simulink model "Vehicle_trailer_FreeModelControl_Modified"  (Simulink 7.7)
settings: Solver=ode3  StartTime=0.0  StopTime=50  FixedStep=Ts  RelTol=1e-3
undefined symbols (not defined in the file): alfa1, BWbaja, Df, jkk, kdf, kif, kpf, L1, L12, L2, manuever, tolerance, v
libraries: simulink x1
settings Model: Creator=Sara  LastModifiedBy=Raul
settings DataIOCC: SignalLoggingSaveFormat=Dataset
settings OptimizationCC: ExpressionDepthLimit=128
settings DebuggingCC: UnderspecifiedInitializationDetection=Simplified  MergeDetectMultiDrivingBlocksExec=error  SolverPrmCheckMsg=none  FcnCallInpInsideContextMsg=Enable All  StateNameClashWarn=none
settings CodeAppCC: CustomSymbolStrType=$N$R$M_T
settings GRTTargetCC: TargetFunctionLibrary=C89/C90 (ANSI)

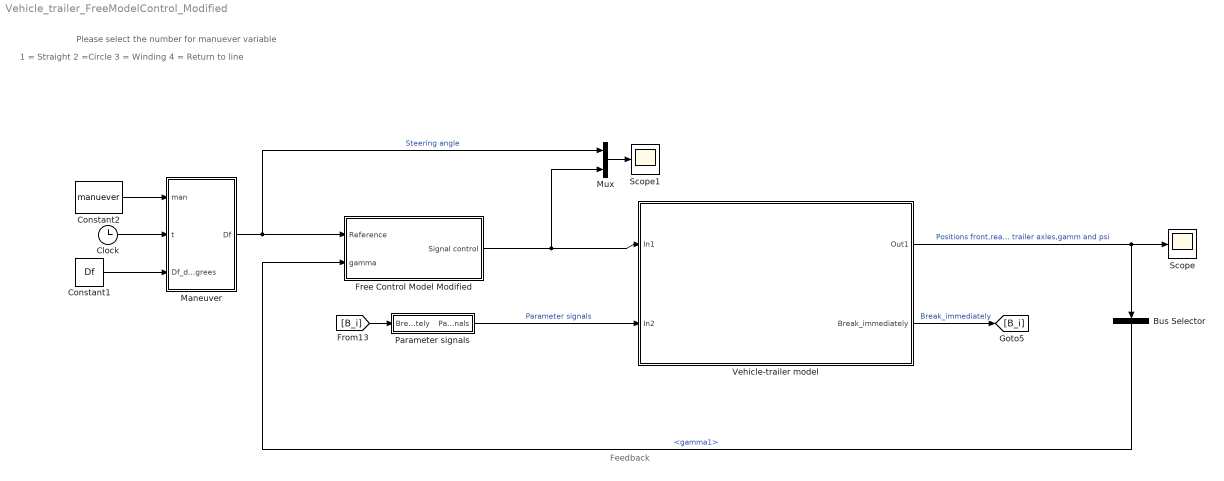
== system Vehicle_trailer_FreeModelControl_Modified ==
  note: 1 = Straight
      | 2 =Circle
      | 3 = Winding
      | 4 = Return to line
  note: Please select the number for manuever variable
  note: Feedback
  Bus Selector : BusSelector  OutputSignals=gamma1
  Clock : Clock
      settings: Decimation=10
  Constant1 : Constant  Value=Df
  Constant2 : Constant  Value=manuever
  Free Control Model Modified : Subsystem
  Maneuver : Stateflow chart  TreatAsAtomicUnit=on
  Mux : Mux  Inputs=2
  Parameter signals : Subsystem
  Scope : Scope
      settings: YMin=-15.4299  YMax=114.11
  Scope1 : Scope
      settings: YMin=-1  YMax=1  SaveName=ScopeData_SteeringAngle
  Vehicle-trailer model : Subsystem
      mask Display: image(imread('vt.png'))
  wires:
  Maneuver/1(Df) -> Mux/1, Free Control Model Modified/1(Reference)  "Steering angle"
  Constant2/1 -> Maneuver/1(man)
  Clock/1 -> Maneuver/2(t)
  Parameter signals/1(Parameter signals) -> Vehicle-trailer model/2(In2)  "Parameter signals"
  Vehicle-trailer model/2(Break_immediately) -> [B_i]  "Break_immediately"
  [B_i] -> Parameter signals/1(Break_immediately)
  Constant1/1 -> Maneuver/3(Df_degrees)
  Free Control Model Modified/1(Signal control) -> Vehicle-trailer model/1(In1), Mux/2
  Bus Selector/1 -> Free Control Model Modified/2(gamma)  "<gamma1>"
  Mux/1 -> Scope1/1
  Vehicle-trailer model/1(Out1) -> Scope/1, Bus Selector/1  "Positions front,rear and trailer axles,gamm and psi"

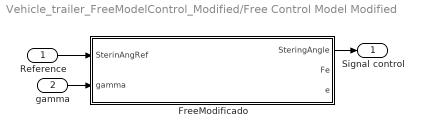
== system Vehicle_trailer_FreeModelControl_Modified/Free Control Model Modified ==
  Reference : Inport
  gamma : Inport  Port=2
  FreeModificado : Subsystem
  Signal control : Outport
  wires:
  Reference/1 -> FreeModificado/1(SterinAngRef)
  FreeModificado/1(SteringAngle) -> Signal control/1
  gamma/1 -> FreeModificado/2(gamma)

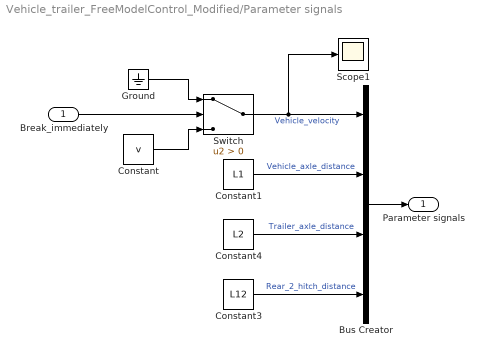
== system Vehicle_trailer_FreeModelControl_Modified/Parameter signals ==
  Break_immediately : Inport
  Bus Creator : BusCreator
  Constant : Constant  Value=v
  Constant1 : Constant  Value=L1
  Constant3 : Constant  Value=L12
  Constant4 : Constant  Value=L2
  Ground : Ground
  Scope1 : Scope
      settings: YMin=-1  YMax=1  SaveName=ScopeData4
  Switch : Switch  Criteria=u2 > Threshold
  Parameter signals : Outport
  wires:
  Constant1/1 -> Bus Creator/2  "Vehicle_axle_distance"
  Constant4/1 -> Bus Creator/3  "Trailer_axle_distance"
  Constant3/1 -> Bus Creator/4  "Rear_2_hitch_distance"
  Bus Creator/1 -> Parameter signals/1
  Switch/1 -> Bus Creator/1, Scope1/1  "Vehicle_velocity"
  Break_immediately/1 -> Switch/2
  Ground/1 -> Switch/1
  Constant/1 -> Switch/3

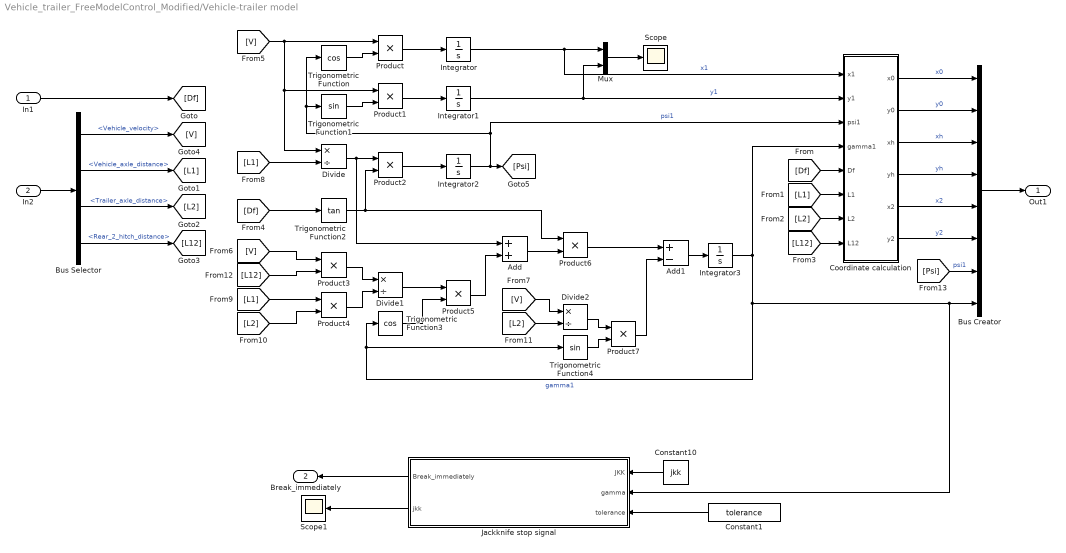
== system Vehicle_trailer_FreeModelControl_Modified/Vehicle-trailer model ==
  In1 : Inport
  In2 : Inport  Port=2
  Add : Sum
  Add1 : Sum  Inputs=+-
  Bus Creator : BusCreator  Inputs=8
  Bus Selector : BusSelector  OutputSignals=Vehicle_velocity,Vehicle_axle_distance,Trailer_axle_distance,Rear_2_hitch_distance
  Constant1 : Constant  Value=tolerance
  Constant10 : Constant  Value=jkk
  Coordinate calculation : Stateflow chart  TreatAsAtomicUnit=on
  Divide : Product  Inputs=*/
  Divide1 : Product  Inputs=*/
  Divide2 : Product  Inputs=*/
  Integrator{,1..3} (4 alike) : Integrator
  "Jackknife stop signal " : Stateflow chart  TreatAsAtomicUnit=on
  Mux : Mux  Inputs=2
  Product{,1..7} (8 alike) : Product
  Scope : Scope
      settings: YMin=-15.0157  YMax=26.5952  SaveName=Car
  Scope1 : Scope
      settings: YMin=-15.0157  YMax=26.5952  SaveName=ScopeData_jkk
  Trigonometric Function : Trigonometry  Operator=cos
  Trigonometric Function1 : Trigonometry
  Trigonometric Function2 : Trigonometry  Operator=tan
  Trigonometric Function3 : Trigonometry  Operator=cos
  Trigonometric Function4 : Trigonometry
  Out1 : Outport
  Break_immediately : Outport  Port=2
  wires:
  Trigonometric Function4/1 -> Product7/2
  Divide2/1 -> Product7/1
  Trigonometric Function1/1 -> Product1/2
  Product1/1 -> Integrator1/1
  Trigonometric Function3/1 -> Product5/2
  Product2/1 -> Integrator2/1
  Divide/1 -> Product2/1, Add/1
  Trigonometric Function2/1 -> Product6/1, Product2/2
  Product6/1 -> Add1/1
  Add1/1 -> Integrator3/1
  Divide1/1 -> Product5/1
  Integrator3/1 -> Trigonometric Function4/1, Trigonometric Function3/1, Bus Creator/8, "Jackknife stop signal "/2(gamma), Coordinate calculation/4(gamma1)  "gamma1"
  Product7/1 -> Add1/2
  Add/1 -> Product6/2
  Product3/1 -> Divide1/1
  Integrator2/1 -> [Psi], Trigonometric Function/1, Trigonometric Function1/1, Coordinate calculation/3(psi1)  "psi1"
  Trigonometric Function/1 -> Product/2
  Product5/1 -> Add/2
  Product4/1 -> Divide1/2
  Product/1 -> Integrator/1
  Integrator/1 -> Coordinate calculation/1(x1), Mux/1  "x1"
  Integrator1/1 -> Mux/2, Coordinate calculation/2(y1)  "y1"
  Mux/1 -> Scope/1
  Bus Creator/1 -> Out1/1
  [Df] -> Coordinate calculation/5(Df)
  [L1] -> Coordinate calculation/6(L1)
  [L2] -> Coordinate calculation/7(L2)
  [L12] -> Coordinate calculation/8(L12)
  [Df] -> Trigonometric Function2/1
  [V] -> Divide/1, Product1/1, Product/1
  [V] -> Product3/1
  [V] -> Divide2/1
  [L1] -> Divide/2
  [L1] -> Product4/1
  [L2] -> Product4/2
  [L2] -> Divide2/2
  [L12] -> Product3/2
  Coordinate calculation/1(x0) -> Bus Creator/1  "x0"
  Coordinate calculation/2(y0) -> Bus Creator/2  "y0"
  [Psi] -> Bus Creator/7  "psi1"
  Coordinate calculation/3(xh) -> Bus Creator/3  "xh"
  Coordinate calculation/4(yh) -> Bus Creator/4  "yh"
  Coordinate calculation/5(x2) -> Bus Creator/5  "x2"
  Coordinate calculation/6(y2) -> Bus Creator/6  "y2"
  In2/1 -> Bus Selector/1
  Bus Selector/1 -> [V]  "<Vehicle_velocity>"
  Bus Selector/2 -> [L1]  "<Vehicle_axle_distance>"
  Bus Selector/3 -> [L2]  "<Trailer_axle_distance>"
  Bus Selector/4 -> [L12]  "<Rear_2_hitch_distance>"
  In1/1 -> [Df]
  Constant10/1 -> "Jackknife stop signal "/1(JKK)
  "Jackknife stop signal "/1(Break_immediately) -> Break_immediately/1
  "Jackknife stop signal "/2(jkk) -> Scope1/1
  Constant1/1 -> "Jackknife stop signal "/3(tolerance)

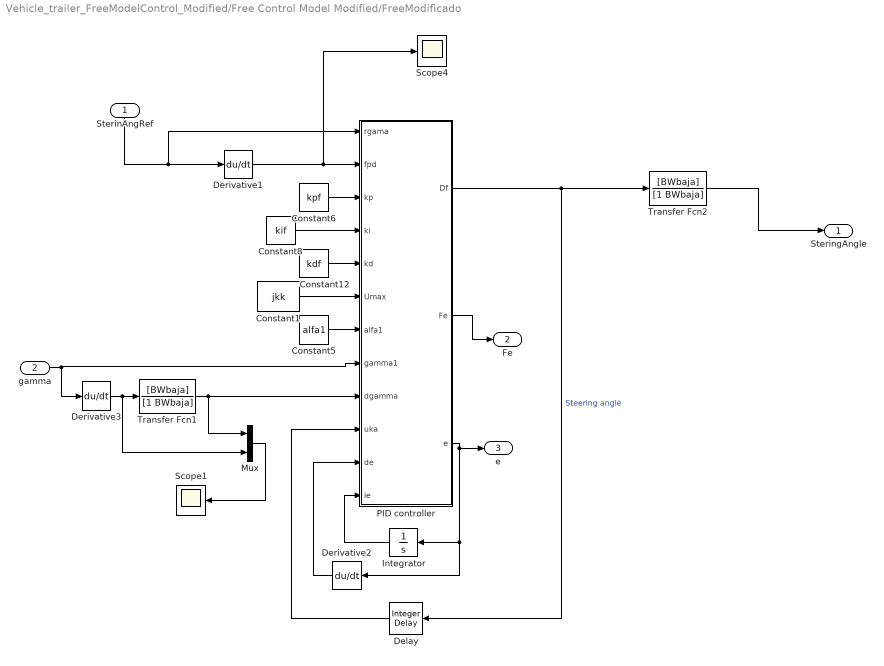
== system Vehicle_trailer_FreeModelControl_Modified/Free Control Model Modified/FreeModificado ==
  SterinAngRef : Inport
  gamma : Inport  Port=2
  Constant1 : Constant  Value=jkk
  Constant12 : Constant  Value=kdf
  Constant5 : Constant  Value=alfa1
  Constant6 : Constant  Value=kpf
  Constant8 : Constant  Value=kif
  Delay : simulink/Discrete/Integer Delay  NumDelays=1  vinit=0  samptime=Ts
  Derivative1 : Derivative
  Derivative2 : Derivative
  Derivative3 : Derivative
  Integrator : Integrator
  Mux : Mux  Inputs=2
  PID controller : Stateflow chart  TreatAsAtomicUnit=on
  Scope1 : Scope
      settings: YMin=-6.82936  YMax=6.54905  SaveName=ScopeData11
  Scope4 : Scope
      settings: YMin=-8750.00000  YMax=8750.00000  SaveName=ScopeData2
  Transfer Fcn1 : TransferFcn  Numerator=[BWbaja]  Denominator=[1 BWbaja]
  Transfer Fcn2 : TransferFcn  Numerator=[BWbaja]  Denominator=[1 BWbaja]
  SteringAngle : Outport
  Fe : Outport  Port=2
  e : Outport  Port=3
  wires:
  Derivative1/1 -> PID controller/2(fpd), Scope4/1
  Constant6/1 -> PID controller/3(kp)
  Constant8/1 -> PID controller/4(ki)
  PID controller/3(e) -> Derivative2/1, Integrator/1, e/1
  Constant5/1 -> PID controller/7(alfa1)
  Delay/1 -> PID controller/10(uka)
  PID controller/2(Fe) -> Fe/1
  Integrator/1 -> PID controller/12(ie)
  Derivative2/1 -> PID controller/11(de)
  PID controller/1(Df) -> Delay/1, Transfer Fcn2/1  "Steering angle"
  Constant12/1 -> PID controller/5(kd)
  SterinAngRef/1 -> Derivative1/1, PID controller/1(rgama)
  Derivative3/1 -> Mux/2, Transfer Fcn1/1
  Transfer Fcn1/1 -> PID controller/9(dgamma), Mux/1
  Mux/1 -> Scope1/1
  gamma/1 -> PID controller/8(gamma1), Derivative3/1
  Constant1/1 -> PID controller/6(Umax)
  Transfer Fcn2/1 -> SteringAngle/1

== matlab function Maneuver ==
  data: man input double; Df output double; t input double; Df_degrees input double
function Df = fcn(man,t,Df_degrees)

switch man
    case 1
        Df=0;
    case 2
        Df=Df_degrees*pi/180;
    case 3
        if t<5
            Df=0;
        elseif (t>=5) && (t<10)
            Df=Df_degrees*pi/180;
        elseif (t>=10) && (t<15)
            Df=0;
        elseif (t>=15) && (t<20)
            Df=-Df_degrees*pi/180;
        elseif (t>=20) && (t<25)
            Df=0;
        else
            Df=Df_degrees*pi/180;
        end
    case 4
        if t<5
            Df=0;
        elseif (t>=5) && (t<10)
            Df=Df_degrees*pi/180;
        else
            Df=0;
        end
    otherwise
        Df=0;
end

== matlab function Vehicle-trailer model/Coordinate calculation ==
  data: x1 input double; x0 output double; y1 input double; psi1 input double; gamma1 input double; Df input double; L1 input double; L2 input double; L12 input double; y0 output double; xh output double; yh output double; x2 output double; y2 output double
function [x0,y0,xh,yh,x2,y2] = fcn(x1,y1,psi1,gamma1,Df,L1,L2,L12)
psi2=psi1-gamma1;
psi0=psi1+Df;

x0=x1+L1*cos(psi1);
y0=y1+L1*sin(psi1);
xh=x1-L12*cos(psi1);
yh=y1-L12*sin(psi1);
x2=x1-L12*cos(psi1)-L2*cos(psi2);
y2=y1-L12*sin(psi1)-L2*sin(psi2);

== matlab function Vehicle-trailer model/Jackknife stop signal  ==
  data: Break_immediately output double; JKK input double; gamma input double; jkk output double; tolerance input double
function [Break_immediately, jkk]= fcn(JKK,gamma,tolerance)
%#codegen

jkk=JKK;

if abs(gamma) > tolerance*jkk 
    Break_immediately=1;
else
    Break_immediately=0;
end

== matlab function Free Control Model Modified/FreeModificado/PID controller ==
  data: rgama input double; fpd input double; kp input double; ki input double; kd input double; Umax input double; alfa1 input double; gamma1 input double; dgamma input double; uka input double; de input double; Df output double; Fe output double; e output double; ie input double
function [Df,Fe,e]= fcn(rgama,fpd,kp,ki,kd,Umax,alfa1,gamma1,dgamma,uka,de,ie)
Fe=dgamma-alfa1*uka;

e=rgama-gamma1;
upi=kp*e+ki*ie+kd*de;
%u=((Fe-fpd)+upi)*1/alfa1;
u=((Fe-fpd))*1/alfa1+upi;
%u=upi;
%Umax=pi/3;
if abs(u)>Umax
    Df=Umax*sign(u);
else
    Df=u;
end
